simulink model "modbusslave_exec"  (Simulink 3.00)
libraries: execlib x6

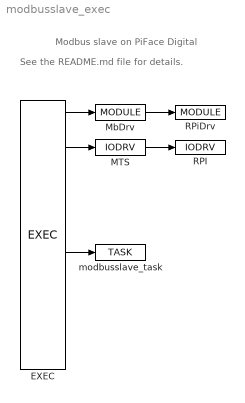
== system modbusslave_exec ==
  note: See the README.md file for details.
  note: Modbus slave on PiFace Digital
  EXEC : execlib/EXEC  target=Generic target device  tick=0.01  ntick0=1  ntick1=50  ntick2=100  ntick3=1200  pri0=5  pri1=9  pri2=13  pri3=18
  MTS : execlib/IODRV  module=MbDrv  classname=MtsDrv  cfgname=modbusslave_iocfg.rio  factor=1  stack=10240  pri=3  timer=off
  MbDrv : execlib/MODULE
  RPI : execlib/IODRV  module=RPiDrv  classname=RPiDrv  factor=1  stack=10240  pri=3  timer=off
  RPiDrv : execlib/MODULE
  modbusslave_task : execlib/TASK  factor=1  start=0  stop=1  stack=10240  MDLOPEN=on
  wires:
  EXEC/1 -> MbDrv/1
  EXEC/2 -> MTS/1
  EXEC/5 -> modbusslave_task/1
  MTS/1 -> RPI/1
  MbDrv/1 -> RPiDrv/1
